simulink model "PID_Insuline_and_Glucogen"  (R2017b)
settings: Solver=ode45  StartTime=0.0  StopTime=18000  RelTol=1e-3
libraries: simulink x5
settings Model: Creator=Nandhini . S  LastModifiedBy=Sunil

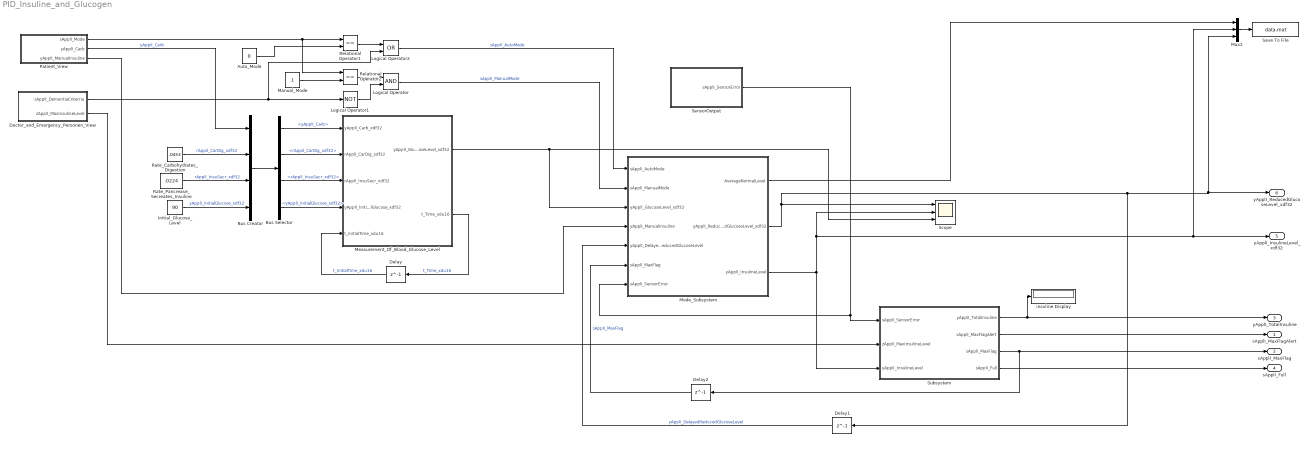
== system PID_Insuline_and_Glucogen ==
  Auto_Mode : Constant  Value=0
  Bus Creator : BusCreator  Inputs=4
  Bus Selector : BusSelector  OutputSignals=yApplI_Carb,rApplI_CarDig_xdf32,rApplI_InsuSecr_xdf32,yApplI_InitialGlucose_xdf32
  Delay : Delay  DelayLength=1  InitialCondition=0  SampleTime=60
  Delay1 : Delay  DelayLength=1  InitialCondition=0  SampleTime=1
  Delay2 : Delay  DelayLength=1  InitialCondition=0  SampleTime=1
  Doctor_and_Emergency_Personen_View : Subsystem
  Initial_Glucose_Level : Constant  Value=90
  Logical Operator : Logic  AllPortsSameDT=off  OutDataTypeStr=boolean
  Logical Operator1 : Logic  Operator=NOT  AllPortsSameDT=off  OutDataTypeStr=boolean
  Logical Operator2 : Logic  Operator=OR  AllPortsSameDT=off  OutDataTypeStr=boolean
  Manual_Mode : Constant
  Measurement_Of_Blood_Glucose_Level : Subsystem
  Mode_Subsystem : Subsystem
  Mux2 : Mux  Inputs=3
  Patient_View : Subsystem
  Rate_Carbohydrates_Digestion : Constant  Value=.0453
  Rate_Pancrease_Secreates_Insuline : Constant  Value=.0224
  Relational Operator1 : RelationalOperator  Operator===  OutDataTypeStr=boolean  RndMeth=Simplest
  Relational Operator2 : RelationalOperator  Operator===  OutDataTypeStr=boolean  RndMeth=Simplest
  Save To File : ToFile  Filename=data.mat  MatrixName=diabetic
  Scope : Scope  NumInputPorts=3
  SensorOutput : Subsystem
  Subsystem : Subsystem
  insuline Display : Display
  sApplI_MaxFlagAlert : Outport
  sApplI_MaxFlag : Outport  Port=2
  yApplI_TotalInsuline : Outport  Port=3
  sApplI_Full : Outport  Port=4
  yApplI_InsulineLevel_xdf32 : Outport  Port=5
  yApplI_ReducedGlucoseLevel_xdf32 : Outport  Port=6  InitialOutput=[0]
  wires:
  Bus Selector/4 -> Measurement_Of_Blood_Glucose_Level/4(yApplI_InitialGlucose_xdf32)  "<yApplI_InitialGlucose_xdf32>"
  Bus Selector/1 -> Measurement_Of_Blood_Glucose_Level/1(yApplI_Carb_xdf32)  "<yApplI_Carb>"
  Bus Creator/1 -> Bus Selector/1
  Bus Selector/2 -> Measurement_Of_Blood_Glucose_Level/2(rApplI_CarDig_xdf32)  "<rApplI_CarDig_xdf32>"
  Initial_Glucose_Level/1 -> Bus Creator/4  "yApplI_InitialGlucose_xdf32"
  Bus Selector/3 -> Measurement_Of_Blood_Glucose_Level/3(rApplI_InsuSecr_xdf32)  "<rApplI_InsuSecr_xdf32>"
  Rate_Pancrease_Secreates_Insuline/1 -> Bus Creator/3  "rApplI_InsuSecr_xdf32"
  Rate_Carbohydrates_Digestion/1 -> Bus Creator/2  "rApplI_CarDig_xdf32"
  Patient_View/2(yApplI_Carb) -> Bus Creator/1  "yApplI_Carb"
  Measurement_Of_Blood_Glucose_Level/1(yApplI_GlucoseLevel_xdf32) -> Mode_Subsystem/3(yApplI_GlucoseLevel_xdf32), Scope/3
  Relational Operator2/1 -> Logical Operator/1
  Auto_Mode/1 -> Relational Operator1/2
  Logical Operator1/1 -> Logical Operator/2
  Manual_Mode/1 -> Relational Operator2/2
  Relational Operator1/1 -> Logical Operator2/1
  Patient_View/1(sApplI_Mode) -> Relational Operator2/1, Relational Operator1/1
  Doctor_and_Emergency_Personen_View/1(sApplI_DementiaCriterria) -> Logical Operator2/2, Logical Operator1/1
  Doctor_and_Emergency_Personen_View/2(zApplI_MaxInsulineLevel) -> Subsystem/2(zApplI_MaxInsulineLevel)
  Subsystem/2(sApplI_MaxFlagAlert) -> sApplI_MaxFlagAlert/1
  Subsystem/3(sApplI_MaxFlag) -> Delay2/1, sApplI_MaxFlag/1
  Logical Operator2/1 -> Mode_Subsystem/1(sApplI_AutoMode)  "sApplI_AutoMode"
  Logical Operator/1 -> Mode_Subsystem/2(sApplI_ManualMode)  "sApplI_ManualMode"
  Patient_View/3(yApplI_ManualInsuline) -> Mode_Subsystem/4(yApplI_ManualInsuline)
  Mode_Subsystem/3(yApplI_InsulineLevel) -> Subsystem/3(yApplI_InsulineLevel), Mux2/2, yApplI_InsulineLevel_xdf32/1, Scope/2
  Mode_Subsystem/2(yApplI_ReducedGlucoseLevel_xdf32) -> Mux2/3, yApplI_ReducedGlucoseLevel_xdf32/1, Delay1/1, Scope/1
  Subsystem/1(yApplI_TotalInsuline) -> insuline Display/1, yApplI_TotalInsuline/1
  Subsystem/4(sApplI_Full) -> sApplI_Full/1
  SensorOutput/1(sApplI_SensorError) -> Mode_Subsystem/7(sApplI_SensorError), Subsystem/1(sApplI_SensorError)
  Mux2/1 -> Save To File/1
  Mode_Subsystem/1(AverageNormalLevel) -> Mux2/1
  Delay1/1 -> Mode_Subsystem/5(yApplI_DelayedReducedGlucoseLevel)  "yApplI_DelayedReducedGlucoseLevel"
  Measurement_Of_Blood_Glucose_Level/2(t_Time_xdu16) -> Delay/1  "t_Time_xdu16"
  Delay/1 -> Measurement_Of_Blood_Glucose_Level/5(t_InitialTime_xdu16)  "t_InitialTime_xdu16"
  Delay2/1 -> Mode_Subsystem/6(sApplI_MaxFlag)  "sApplI_MaxFlag"

== system PID_Insuline_and_Glucogen/Doctor_and_Emergency_Personen_View ==
  Dementia_Criteria : Constant  Value=0
  Man_Insuline_Level : Constant  Value=30000
  sApplI_DementiaCriterria : Outport
  zApplI_MaxInsulineLevel : Outport  Port=2
  wires:
  Dementia_Criteria/1 -> sApplI_DementiaCriterria/1  "sApplI_DementiaCriterria"
  Man_Insuline_Level/1 -> zApplI_MaxInsulineLevel/1  "zApplI_MaxInsulineLevel"

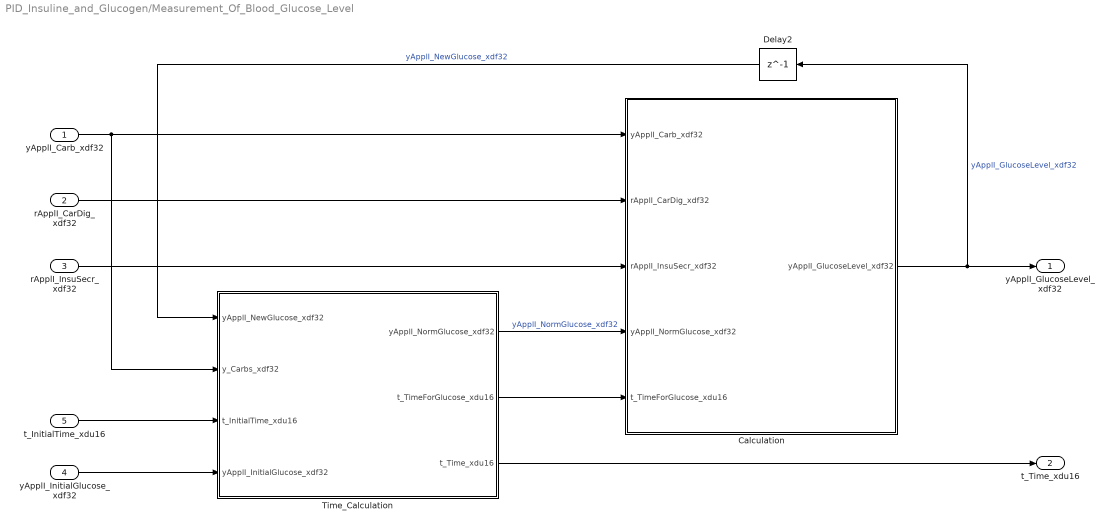
== system PID_Insuline_and_Glucogen/Measurement_Of_Blood_Glucose_Level ==
  yApplI_Carb_xdf32 : Inport
  rApplI_CarDig_xdf32 : Inport  Port=2
  rApplI_InsuSecr_xdf32 : Inport  Port=3
  yApplI_InitialGlucose_xdf32 : Inport  Port=4
  t_InitialTime_xdu16 : Inport  Port=5
  Calculation : Subsystem
  Delay2 : Delay  DelayLength=1  InitialCondition=0  SampleTime=60
  Time_Calculation : Subsystem
  yApplI_GlucoseLevel_xdf32 : Outport
  t_Time_xdu16 : Outport  Port=2
  wires:
  yApplI_Carb_xdf32/1 -> Calculation/1(yApplI_Carb_xdf32), Time_Calculation/2(y_Carbs_xdf32)
  rApplI_CarDig_xdf32/1 -> Calculation/2(rApplI_CarDig_xdf32)
  rApplI_InsuSecr_xdf32/1 -> Calculation/3(rApplI_InsuSecr_xdf32)
  t_InitialTime_xdu16/1 -> Time_Calculation/3(t_InitialTime_xdu16)
  Time_Calculation/3(t_Time_xdu16) -> t_Time_xdu16/1
  Calculation/1(yApplI_GlucoseLevel_xdf32) -> Delay2/1, yApplI_GlucoseLevel_xdf32/1  "yApplI_GlucoseLevel_xdf32"
  Delay2/1 -> Time_Calculation/1(yApplI_NewGlucose_xdf32)  "yApplI_NewGlucose_xdf32"
  Time_Calculation/2(t_TimeForGlucose_xdu16) -> Calculation/5(t_TimeForGlucose_xdu16)
  yApplI_InitialGlucose_xdf32/1 -> Time_Calculation/4(yApplI_InitialGlucose_xdf32)
  Time_Calculation/1(yApplI_NormGlucose_xdf32) -> Calculation/4(yApplI_NormGlucose_xdf32)  "yApplI_NormGlucose_xdf32"

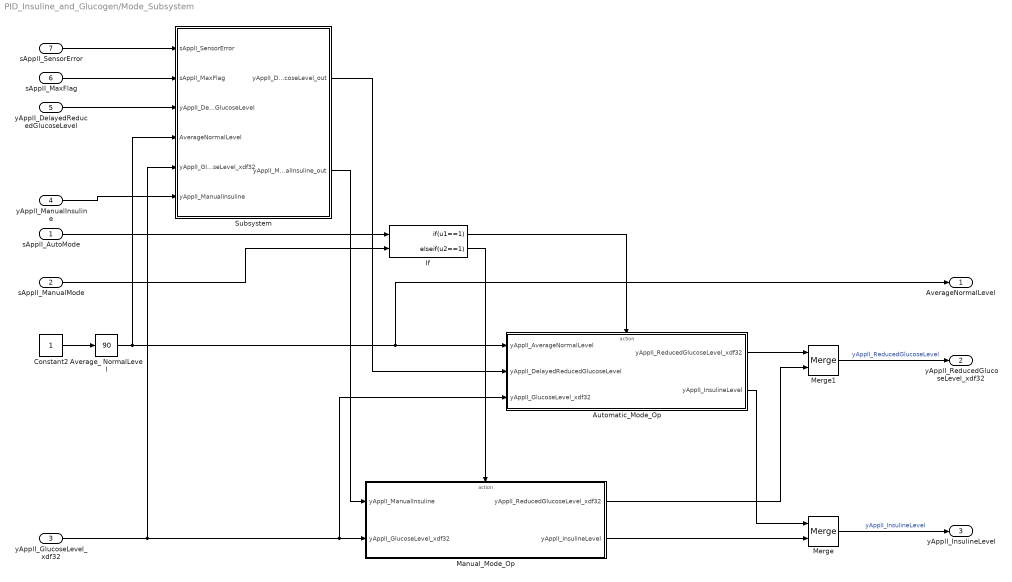
== system PID_Insuline_and_Glucogen/Mode_Subsystem ==
  sApplI_AutoMode : Inport
  sApplI_ManualMode : Inport  Port=2
  yApplI_GlucoseLevel_xdf32 : Inport  Port=3
  yApplI_ManualInsuline : Inport  Port=4
  yApplI_DelayedReducedGlucoseLevel : Inport  Port=5
  sApplI_MaxFlag : Inport  Port=6
  sApplI_SensorError : Inport  Port=7
  Automatic_Mode_Op : Subsystem
  Average_ NormalLevel : simulink/Math Operations/Slider Gain  gain=90  low=50  high=120
  Constant2 : Constant
  If : If  NumInputs=2  IfExpression=u1==1  ElseIfExpressions=u2==1  ShowElse=off  ZeroCross=off
  Manual_Mode_Op : Subsystem
  Merge : Merge
  Merge1 : Merge
  Subsystem : Subsystem
  AverageNormalLevel : Outport
  yApplI_ReducedGlucoseLevel_xdf32 : Outport  Port=2
  yApplI_InsulineLevel : Outport  Port=3
  wires:
  yApplI_GlucoseLevel_xdf32/1 -> Subsystem/5(yApplI_GlucoseLevel_xdf32), Automatic_Mode_Op/3(yApplI_GlucoseLevel_xdf32), Manual_Mode_Op/2(yApplI_GlucoseLevel_xdf32)
  Average_ NormalLevel/1 -> Subsystem/4(AverageNormalLevel), AverageNormalLevel/1, Automatic_Mode_Op/1(yApplI_AverageNormalLevel)
  sApplI_ManualMode/1 -> If/2
  Merge1/1 -> yApplI_ReducedGlucoseLevel_xdf32/1  "yApplI_ReducedGlucoseLevel"
  Automatic_Mode_Op/1(yApplI_ReducedGlucoseLevel_xdf32) -> Merge1/1
  Manual_Mode_Op/1(yApplI_ReducedGlucoseLevel_xdf32) -> Merge1/2
  If/2 -> Manual_Mode_Op/Action
  Manual_Mode_Op/2(yApplI_InsulineLevel) -> Merge/2
  If/1 -> Automatic_Mode_Op/Action
  Automatic_Mode_Op/2(yApplI_InsulineLevel) -> Merge/1
  Merge/1 -> yApplI_InsulineLevel/1  "yApplI_InsulineLevel"
  yApplI_ManualInsuline/1 -> Subsystem/6(yApplI_ManualInsuline)
  Constant2/1 -> Average_ NormalLevel/1
  yApplI_DelayedReducedGlucoseLevel/1 -> Subsystem/3(yApplI_DelayedReducedGlucoseLevel)
  sApplI_AutoMode/1 -> If/1
  sApplI_SensorError/1 -> Subsystem/1(sApplI_SensorError)
  sApplI_MaxFlag/1 -> Subsystem/2(sApplI_MaxFlag)
  Subsystem/1(yApplI_DelayedReducedGlucoseLevel_out) -> Automatic_Mode_Op/2(yApplI_DelayedReducedGlucoseLevel)
  Subsystem/2(yApplI_ManualInsuline_out) -> Manual_Mode_Op/1(yApplI_ManualInsuline)

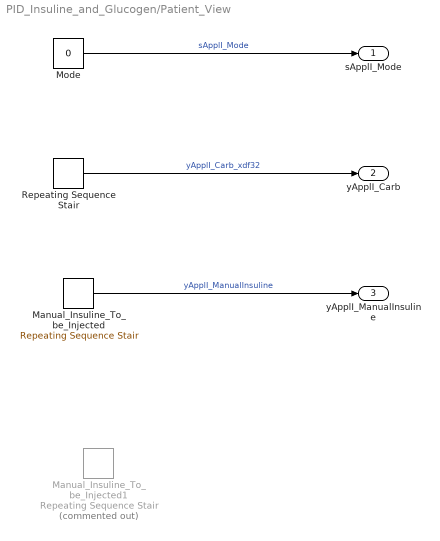
== system PID_Insuline_and_Glucogen/Patient_View ==
  Manual_Insuline_To_be_Injected : simulink/Sources/Repeating Sequence Stair  OutValues="[10 0 0 0  10 0 0 0 0 0 0 0 0 0 10 0 0 ].'"  tsamp=1000  OutMin=[]  OutMax=[]  OutDataTypeStr=double  OutputDataTypeScalingMode=double  OutDataType=fixdt(0,8)  ConRadixGroup=Best Precision: Vector-wise  OutScaling=2^-12
  Manual_Insuline_To_be_Injected1 : simulink/Sources/Repeating Sequence Stair  Commented=on  OutValues=[1 0 0 0 1 1 0 0 0 0 1 1 0 0 0 1 0 0 ].'  tsamp=1000  OutMin=[]  OutMax=[]  OutDataTypeStr=double  OutputDataTypeScalingMode=double  OutDataType=fixdt(0,8)  ConRadixGroup=Best Precision: Vector-wise  OutScaling=2^-12
  Mode : Constant  Value=0
  Repeating Sequence Stair : simulink/Sources/Repeating Sequence Stair  OutValues=[500 40 200 210 300 160].'  tsamp=3000  OutMin=[]  OutMax=[]  OutDataTypeStr=double  OutputDataTypeScalingMode=double  OutDataType=fixdt(0,8)  ConRadixGroup=Best Precision: Vector-wise  OutScaling=2^-12
  sApplI_Mode : Outport
  yApplI_Carb : Outport  Port=2
  yApplI_ManualInsuline : Outport  Port=3
  wires:
  Mode/1 -> sApplI_Mode/1  "sApplI_Mode"
  Repeating Sequence Stair/1 -> yApplI_Carb/1  "yApplI_Carb_xdf32"
  Manual_Insuline_To_be_Injected/1 -> yApplI_ManualInsuline/1  "yApplI_ManualInsuline"

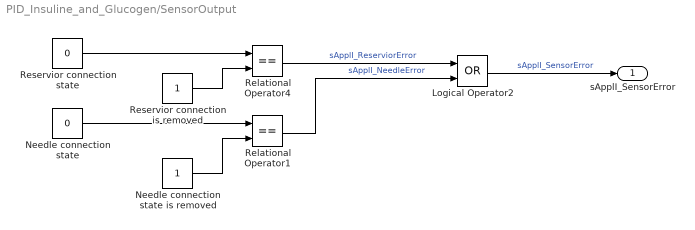
== system PID_Insuline_and_Glucogen/SensorOutput ==
  Logical Operator2 : Logic  Operator=OR  AllPortsSameDT=off  OutDataTypeStr=boolean
  Needle connection state : Constant  Value=0
  Needle connection state is removed : Constant
  Relational Operator1 : RelationalOperator  Operator===  OutDataTypeStr=boolean  RndMeth=Simplest
  Relational Operator4 : RelationalOperator  Operator===  OutDataTypeStr=boolean  RndMeth=Simplest
  Reservior connection is removed : Constant
  Reservior connection state : Constant  Value=0
  sApplI_SensorError : Outport
  wires:
  Reservior connection state/1 -> Relational Operator4/1
  Reservior connection is removed/1 -> Relational Operator4/2
  Needle connection state/1 -> Relational Operator1/1
  Needle connection state is removed/1 -> Relational Operator1/2
  Relational Operator4/1 -> Logical Operator2/1  "sApplI_ReserviorError"
  Relational Operator1/1 -> Logical Operator2/2  "sApplI_NeedleError"
  Logical Operator2/1 -> sApplI_SensorError/1  "sApplI_SensorError"

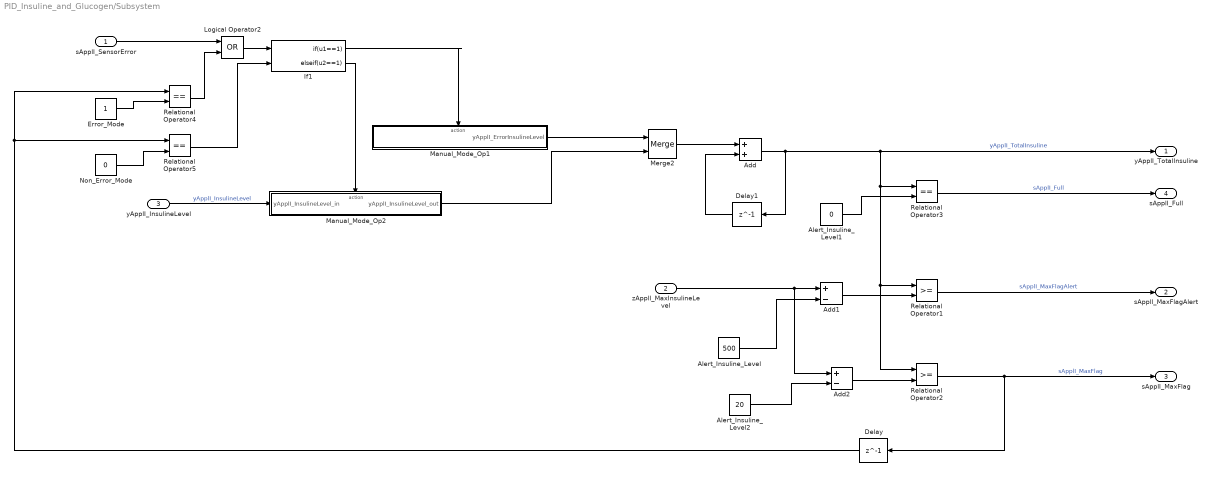
== system PID_Insuline_and_Glucogen/Subsystem ==
  sApplI_SensorError : Inport
  zApplI_MaxInsulineLevel : Inport  Port=2
  yApplI_InsulineLevel : Inport  Port=3
  Add : Sum
  Add1 : Sum  Inputs=+-
  Add2 : Sum  Inputs=+-
  Alert_Insuline_Level : Constant  Value=500
  Alert_Insuline_Level1 : Constant  Value=0
  Alert_Insuline_Level2 : Constant  Value=20
  Delay : Delay  DelayLength=1  InitialCondition=0
  Delay1 : Delay  DelayLength=1  InitialCondition=0  SampleTime=1
  Error_Mode : Constant
  If1 : If  NumInputs=2  IfExpression=u1==1  ElseIfExpressions=u2==1  ShowElse=off
  Logical Operator2 : Logic  Operator=OR  AllPortsSameDT=off  OutDataTypeStr=boolean
  Manual_Mode_Op1 : Subsystem
  Manual_Mode_Op2 : Subsystem
  Merge2 : Merge
  Non_Error_Mode : Constant  Value=0
  Relational Operator1 : RelationalOperator  OutDataTypeStr=boolean  RndMeth=Simplest
  Relational Operator2 : RelationalOperator  OutDataTypeStr=boolean  RndMeth=Simplest
  Relational Operator3 : RelationalOperator  Operator===  OutDataTypeStr=boolean  RndMeth=Simplest
  Relational Operator4 : RelationalOperator  Operator===  OutDataTypeStr=boolean  RndMeth=Simplest
  Relational Operator5 : RelationalOperator  Operator===  OutDataTypeStr=boolean  RndMeth=Simplest
  yApplI_TotalInsuline : Outport
  sApplI_MaxFlagAlert : Outport  Port=2
  sApplI_MaxFlag : Outport  Port=3
  sApplI_Full : Outport  Port=4
  wires:
  Delay1/1 -> Add/2
  Add/1 -> Delay1/1, Relational Operator3/1, Relational Operator2/1, Relational Operator1/1, yApplI_TotalInsuline/1  "yApplI_TotalInsuline"
  Merge2/1 -> Add/1
  zApplI_MaxInsulineLevel/1 -> Add2/1, Add1/1
  Alert_Insuline_Level/1 -> Add1/2
  Add1/1 -> Relational Operator1/2
  Relational Operator1/1 -> sApplI_MaxFlagAlert/1  "sApplI_MaxFlagAlert"
  Relational Operator2/1 -> Delay/1, sApplI_MaxFlag/1  "sApplI_MaxFlag"
  Alert_Insuline_Level1/1 -> Relational Operator3/2
  Relational Operator3/1 -> sApplI_Full/1  "sApplI_Full"
  Relational Operator5/1 -> If1/2
  Error_Mode/1 -> Relational Operator4/2
  Relational Operator4/1 -> Logical Operator2/2
  Delay/1 -> Relational Operator5/1, Relational Operator4/1
  Non_Error_Mode/1 -> Relational Operator5/2
  If1/1 -> Manual_Mode_Op1/Action
  If1/2 -> Manual_Mode_Op2/Action
  Manual_Mode_Op1/1(yApplI_ErrorInsulineLevel) -> Merge2/1
  yApplI_InsulineLevel/1 -> Manual_Mode_Op2/1(yApplI_InsulineLevel_in)  "yApplI_InsulineLevel"
  Manual_Mode_Op2/1(yApplI_InsulineLevel_out) -> Merge2/2
  Logical Operator2/1 -> If1/1
  sApplI_SensorError/1 -> Logical Operator2/1
  Alert_Insuline_Level2/1 -> Add2/2
  Add2/1 -> Relational Operator2/2

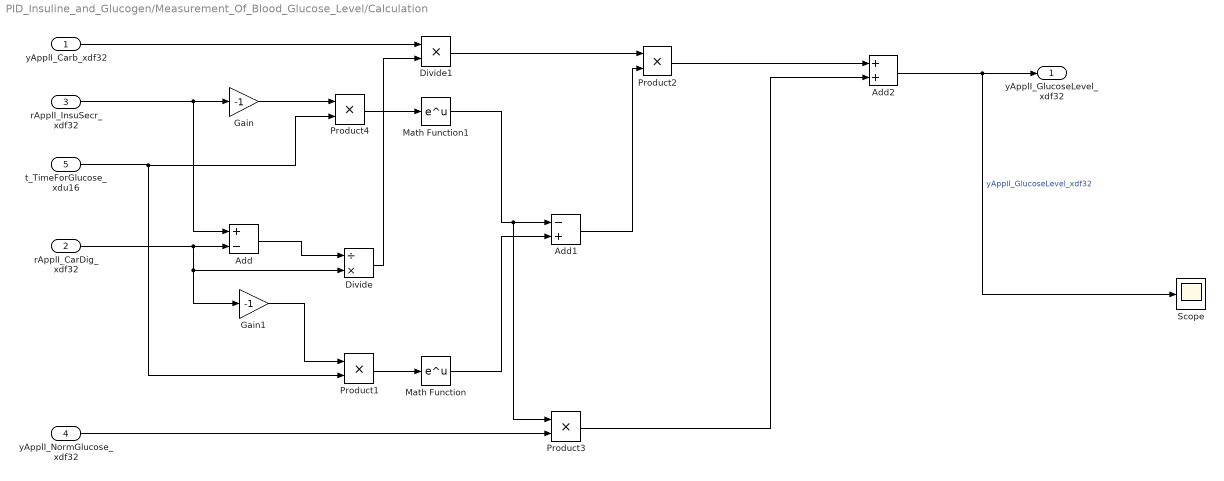
== system PID_Insuline_and_Glucogen/Measurement_Of_Blood_Glucose_Level/Calculation ==
  yApplI_Carb_xdf32 : Inport
  rApplI_CarDig_xdf32 : Inport  Port=2
  rApplI_InsuSecr_xdf32 : Inport  Port=3
  yApplI_NormGlucose_xdf32 : Inport  Port=4
  t_TimeForGlucose_xdu16 : Inport  Port=5
  Add : Sum  Inputs=+-
  Add1 : Sum  Inputs=-+  OutDataTypeStr=double
  Add2 : Sum
  Divide : Product  Inputs=/*
  Divide1 : Product  Inputs=**
  Gain : Gain  Gain=-1
  Gain1 : Gain  Gain=-1
  Math Function : Math  SaturateOnIntegerOverflow=on
  Math Function1 : Math  SaturateOnIntegerOverflow=on
  Product{1..4} (4 alike) : Product
  Scope : Scope
  yApplI_GlucoseLevel_xdf32 : Outport
  wires:
  rApplI_CarDig_xdf32/1 -> Add/2, Gain1/1, Divide/2
  rApplI_InsuSecr_xdf32/1 -> Add/1, Gain/1
  yApplI_NormGlucose_xdf32/1 -> Product3/2
  yApplI_Carb_xdf32/1 -> Divide1/1
  Add/1 -> Divide/1
  Divide/1 -> Divide1/2
  Gain1/1 -> Product1/1
  t_TimeForGlucose_xdu16/1 -> Product4/2, Product1/2
  Gain/1 -> Product4/1
  Product1/1 -> Math Function/1
  Math Function1/1 -> Product3/1, Add1/1
  Math Function/1 -> Add1/2
  Add1/1 -> Product2/2
  Divide1/1 -> Product2/1
  Product2/1 -> Add2/1
  Add2/1 -> Scope/1, yApplI_GlucoseLevel_xdf32/1  "yApplI_GlucoseLevel_xdf32"
  Product4/1 -> Math Function1/1
  Product3/1 -> Add2/2

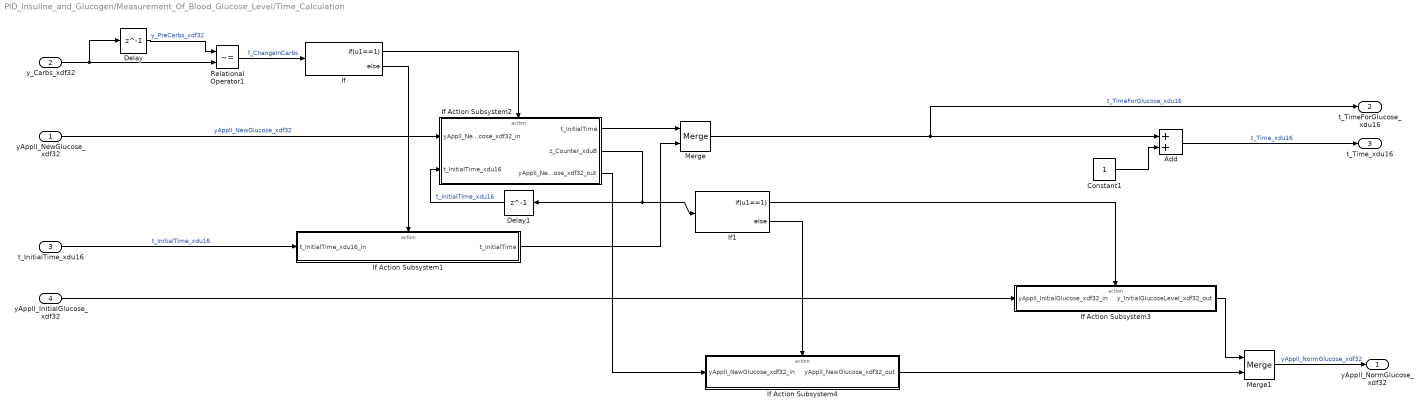
== system PID_Insuline_and_Glucogen/Measurement_Of_Blood_Glucose_Level/Time_Calculation ==
  yApplI_NewGlucose_xdf32 : Inport
  y_Carbs_xdf32 : Inport  Port=2
  t_InitialTime_xdu16 : Inport  Port=3
  yApplI_InitialGlucose_xdf32 : Inport  Port=4
  Add : Sum
  Constant1 : Constant
  Delay : Delay  DelayLength=1  InitialCondition=0  SampleTime=60
  Delay1 : Delay  DelayLength=1  InitialCondition=0  SampleTime=60
  If : If  IfExpression=u1==1
  If Action Subsystem1 : Subsystem  TreatAsAtomicUnit=on
  If Action Subsystem2 : Subsystem  TreatAsAtomicUnit=on
  If Action Subsystem3 : Subsystem  TreatAsAtomicUnit=on
  If Action Subsystem4 : Subsystem  TreatAsAtomicUnit=on
  If1 : If  IfExpression=u1==1
  Merge : Merge
  Merge1 : Merge
  Relational Operator1 : RelationalOperator  Operator=~=  OutDataTypeStr=boolean  RndMeth=Simplest
  yApplI_NormGlucose_xdf32 : Outport
  t_TimeForGlucose_xdu16 : Outport  Port=2
  t_Time_xdu16 : Outport  Port=3
  wires:
  If/2 -> If Action Subsystem1/Action
  Merge/1 -> Add/1, t_TimeForGlucose_xdu16/1  "t_TimeForGlucose_xdu16"
  t_InitialTime_xdu16/1 -> If Action Subsystem1/1(t_InitialTime_xdu16_in)  "t_InitialTime_xdu16"
  y_Carbs_xdf32/1 -> Delay/1, Relational Operator1/2
  Delay/1 -> Relational Operator1/1  "y_PreCarbs_xdf32"
  If/1 -> If Action Subsystem2/Action
  If Action Subsystem2/1(t_InitialTime) -> Merge/1
  Constant1/1 -> Add/2
  Add/1 -> t_Time_xdu16/1  "t_Time_xdu16"
  If Action Subsystem1/1(t_InitialTime) -> Merge/2
  Relational Operator1/1 -> If/1  "f_ChangeInCarbs"
  If Action Subsystem2/2(z_Counter_xdu8) -> Delay1/1, If1/1
  Delay1/1 -> If Action Subsystem2/2(t_InitialTime_xdu16)  "t_InitialTime_xdu16"
  If1/1 -> If Action Subsystem3/Action
  If1/2 -> If Action Subsystem4/Action
  yApplI_InitialGlucose_xdf32/1 -> If Action Subsystem3/1(yApplI_InitialGlucose_xdf32_in)
  If Action Subsystem3/1(y_InitialGlucoseLevel_xdf32_out) -> Merge1/1
  Merge1/1 -> yApplI_NormGlucose_xdf32/1  "yApplI_NormGlucose_xdf32"
  If Action Subsystem2/3(yApplI_NewGlucose_xdf32_out) -> If Action Subsystem4/1(yApplI_NewGlucose_xdf32_in)
  yApplI_NewGlucose_xdf32/1 -> If Action Subsystem2/1(yApplI_NewGlucose_xdf32_in)  "yApplI_NewGlucose_xdf32"
  If Action Subsystem4/1(yApplI_NewGlucose_xdf32_out) -> Merge1/2

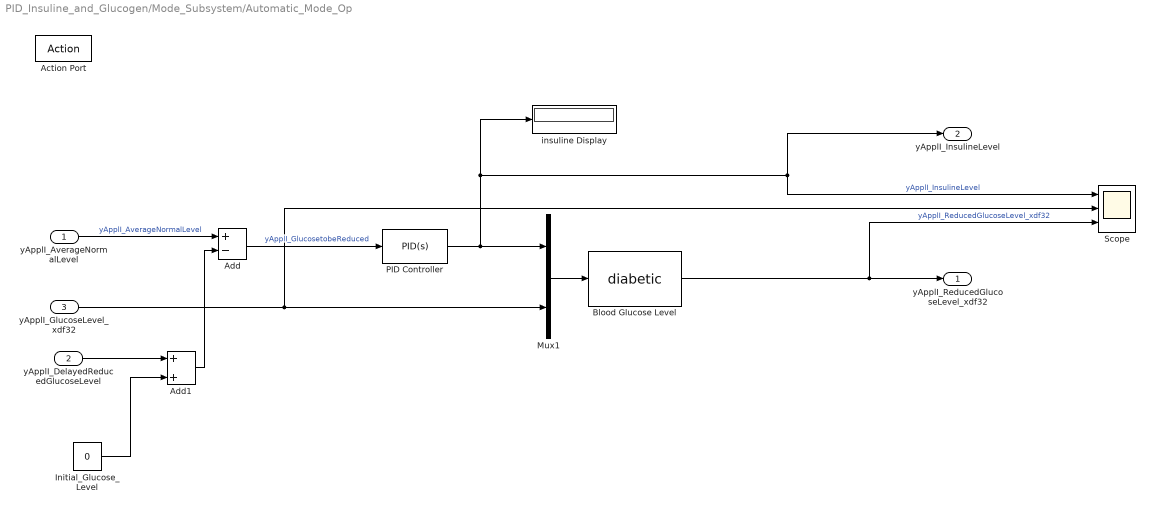
== system PID_Insuline_and_Glucogen/Mode_Subsystem/Automatic_Mode_Op ==
  yApplI_AverageNormalLevel : Inport
  yApplI_DelayedReducedGlucoseLevel : Inport  Port=2
  yApplI_GlucoseLevel_xdf32 : Inport  Port=3
  Action Port : ActionPort  ActionType=then
  Add : Sum  Inputs=+-
  Add1 : Sum
  Blood Glucose Level : S-Function  FunctionName=diabetic  SFunctionDeploymentMode=off  EnableBusSupport=off
  Initial_Glucose_Level : Constant  Value=0
  Mux1 : Mux  Inputs=2
  PID Controller : simulink/Continuous/PID Controller  Controller=PID  TimeDomain=Continuous-time  SampleTime=-1  IntegratorMethod=Forward Euler  FilterMethod=Forward Euler  Form=Parallel  UseFilter=on  ControllerParametersSource=internal  P=-0.05  I=-0.1  D=0  N=100  InitialConditionSource=internal  InitialConditionForIntegrator=3  InitialConditionForFilter=0  ExternalReset=none  LimitOutput=on  UpperSaturationLimit=10  LowerSaturationLimit=0  LinearizeAsGain=on  AntiWindupMode=back-calculation  Kb=1  TrackingMode=off  Kt=1  PParamMin=[]  PParamMax=[]  IParamMin=[]  IParamMax=[]  DParamMin=[]  DParamMax=[]  NParamMin=[]  NParamMax=[]  KbParamMin=[]  KbParamMax=[]  KtParamMin=[]  KtParamMax=[]  POutMin=[]  POutMax=[]  IOutMin=[]  IOutMax=[]  DOutMin=[]  DOutMax=[]  NOutMin=[]  NOutMax=[]  KbOutMin=[]  KbOutMax=[]  KtOutMin=[]  KtOutMax=[]  IntegratorOutMin=[]  IntegratorOutMax=[]  FilterOutMin=[]  FilterOutMax=[]  SumOutMin=[]  SumOutMax=[]  SumI1OutMin=[]  SumI1OutMax=[]  SumI2OutMin=[]  SumI2OutMax=[]  SumI3OutMin=[]  SumI3OutMax=[]  SumDOutMin=[]  SumDOutMax=[]  SaturationOutMin=[]  SaturationOutMax=[]  IntegratorContinuousStateAttributes=''  IntegratorStateMustResolveToSignalObject=off  IntegratorRTWStateStorageClass=Auto  FilterContinuousStateAttributes=''  FilterStateMustResolveToSignalObject=off  FilterRTWStateStorageClass=Auto  DifferentiatorICPrevScaledInput=0  DifferentiatorOutMin=[]  DifferentiatorOutMax=[]  InitialConditionSetting=State (most efficient)  FilterDiffOutCoefMin=[]  FilterDiffOutCoefMax=[]  SumDenOutMin=[]  SumDenOutMax=[]  SumNumOutMin=[]  SumNumOutMax=[]  ReciprocalOutMin=[]  ReciprocalOutMax=[]  DivideOutMin=[]  DivideOutMax=[]  TunerSelectOption=Transfer Function Based (PID Tuner App)
  Scope : Scope  NumInputPorts=3
  insuline Display : Display
  yApplI_ReducedGlucoseLevel_xdf32 : Outport  InitialOutput=[0]
  yApplI_InsulineLevel : Outport  Port=2
  wires:
  yApplI_GlucoseLevel_xdf32/1 -> Scope/2, Mux1/2
  yApplI_AverageNormalLevel/1 -> Add/1  "yApplI_AverageNormalLevel"
  Add/1 -> PID Controller/1  "yApplI_GlucosetobeReduced"
  Mux1/1 -> Blood Glucose Level/1
  PID Controller/1 -> yApplI_InsulineLevel/1, Scope/1, insuline Display/1, Mux1/1  "yApplI_InsulineLevel"
  Blood Glucose Level/1 -> yApplI_ReducedGlucoseLevel_xdf32/1, Scope/3  "yApplI_ReducedGlucoseLevel_xdf32"
  Initial_Glucose_Level/1 -> Add1/2
  Add1/1 -> Add/2
  yApplI_DelayedReducedGlucoseLevel/1 -> Add1/1

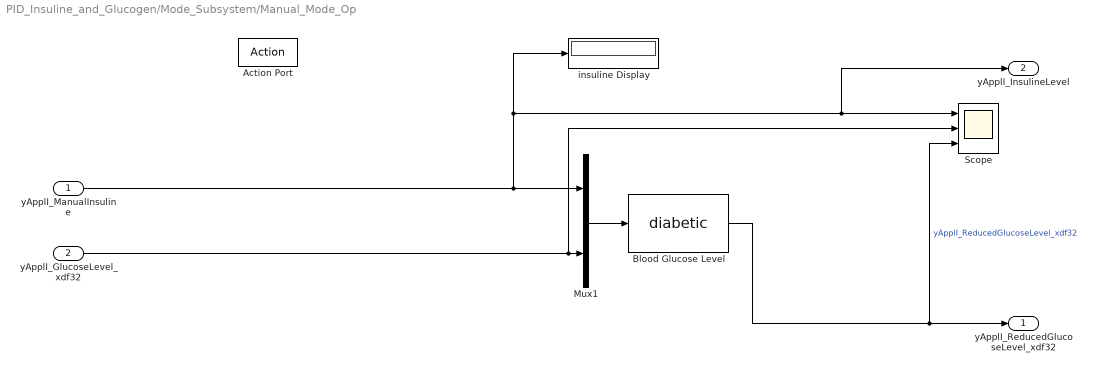
== system PID_Insuline_and_Glucogen/Mode_Subsystem/Manual_Mode_Op ==
  yApplI_ManualInsuline : Inport
  yApplI_GlucoseLevel_xdf32 : Inport  Port=2
  Action Port : ActionPort  ActionType=elseif
  Blood Glucose Level : S-Function  FunctionName=diabetic  SFunctionDeploymentMode=off  EnableBusSupport=off
  Mux1 : Mux  Inputs=2
  Scope : Scope  NumInputPorts=3
  insuline Display : Display
  yApplI_ReducedGlucoseLevel_xdf32 : Outport  InitialOutput=[0]
  yApplI_InsulineLevel : Outport  Port=2
  wires:
  yApplI_GlucoseLevel_xdf32/1 -> Mux1/2, Scope/2
  Mux1/1 -> Blood Glucose Level/1
  yApplI_ManualInsuline/1 -> yApplI_InsulineLevel/1, Scope/1, insuline Display/1, Mux1/1
  Blood Glucose Level/1 -> yApplI_ReducedGlucoseLevel_xdf32/1, Scope/3  "yApplI_ReducedGlucoseLevel_xdf32"

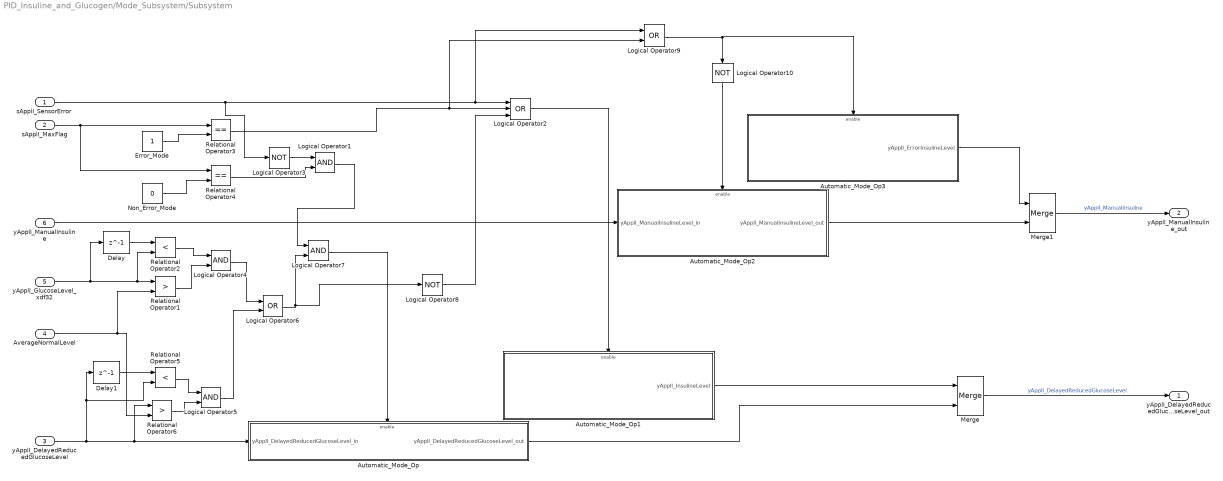
== system PID_Insuline_and_Glucogen/Mode_Subsystem/Subsystem ==
  sApplI_SensorError : Inport
  sApplI_MaxFlag : Inport  Port=2
  yApplI_DelayedReducedGlucoseLevel : Inport  Port=3
  AverageNormalLevel : Inport  Port=4
  yApplI_GlucoseLevel_xdf32 : Inport  Port=5
  yApplI_ManualInsuline : Inport  Port=6
  Automatic_Mode_Op : Subsystem
  Automatic_Mode_Op1 : Subsystem
  Automatic_Mode_Op2 : Subsystem
  Automatic_Mode_Op3 : Subsystem
  Delay : Delay  DelayLength=1  InitialCondition=0  SampleTime=60
  Delay1 : Delay  DelayLength=1  InitialCondition=0  SampleTime=60
  Error_Mode : Constant
  Logical Operator{1,4..5,7} (4 alike) : Logic  AllPortsSameDT=off  OutDataTypeStr=boolean
  Logical Operator10 : Logic  Operator=NOT  AllPortsSameDT=off  OutDataTypeStr=boolean
  Logical Operator2 : Logic  Operator=OR  Inputs=3  AllPortsSameDT=off  OutDataTypeStr=boolean
  Logical Operator3 : Logic  Operator=NOT  AllPortsSameDT=off  OutDataTypeStr=boolean
  Logical Operator6 : Logic  Operator=OR  AllPortsSameDT=off  OutDataTypeStr=boolean
  Logical Operator8 : Logic  Operator=NOT  AllPortsSameDT=off  OutDataTypeStr=boolean
  Logical Operator9 : Logic  Operator=OR  AllPortsSameDT=off  OutDataTypeStr=boolean
  Merge : Merge
  Merge1 : Merge
  Non_Error_Mode : Constant  Value=0
  Relational Operator1 : RelationalOperator  Operator=>  OutDataTypeStr=boolean  RndMeth=Simplest
  Relational Operator2 : RelationalOperator  Operator=<  OutDataTypeStr=boolean  RndMeth=Simplest
  Relational Operator3 : RelationalOperator  Operator===  OutDataTypeStr=boolean  RndMeth=Simplest
  Relational Operator4 : RelationalOperator  Operator===  OutDataTypeStr=boolean  RndMeth=Simplest
  Relational Operator5 : RelationalOperator  Operator=<  OutDataTypeStr=boolean  RndMeth=Simplest
  Relational Operator6 : RelationalOperator  Operator=>  OutDataTypeStr=boolean  RndMeth=Simplest
  yApplI_DelayedReducedGlucoseLevel_out : Outport
  yApplI_ManualInsuline_out : Outport  Port=2
  wires:
  Relational Operator3/1 -> Logical Operator9/2, Logical Operator2/2
  Non_Error_Mode/1 -> Relational Operator4/2
  sApplI_SensorError/1 -> Logical Operator3/1, Logical Operator9/1, Logical Operator2/1
  sApplI_MaxFlag/1 -> Relational Operator4/1, Relational Operator3/1
  Error_Mode/1 -> Relational Operator3/2
  yApplI_DelayedReducedGlucoseLevel/1 -> Relational Operator5/2, Delay1/1, Relational Operator6/1, Automatic_Mode_Op/1(yApplI_DelayedReducedGlucoseLevel_in)
  Relational Operator4/1 -> Logical Operator1/2
  Logical Operator2/1 -> Automatic_Mode_Op1/Enable
  Automatic_Mode_Op1/1(yApplI_InsulineLevel) -> Merge/1
  Automatic_Mode_Op/1(yApplI_DelayedReducedGlucoseLevel_out) -> Merge/2
  Merge/1 -> yApplI_DelayedReducedGlucoseLevel_out/1  "yApplI_DelayedReducedGlucoseLevel"
  Logical Operator3/1 -> Logical Operator1/1
  Logical Operator1/1 -> Logical Operator7/1
  yApplI_GlucoseLevel_xdf32/1 -> Delay/1, Relational Operator2/2, Relational Operator1/1
  AverageNormalLevel/1 -> Relational Operator6/2, Relational Operator1/2
  Delay/1 -> Relational Operator2/1
  Relational Operator2/1 -> Logical Operator4/1
  Relational Operator1/1 -> Logical Operator4/2
  Delay1/1 -> Relational Operator5/1
  Relational Operator5/1 -> Logical Operator5/1
  Relational Operator6/1 -> Logical Operator5/2
  Logical Operator4/1 -> Logical Operator6/1
  Logical Operator5/1 -> Logical Operator6/2
  Logical Operator6/1 -> Logical Operator8/1, Logical Operator7/2
  Logical Operator7/1 -> Automatic_Mode_Op/Enable
  Logical Operator8/1 -> Logical Operator2/3
  yApplI_ManualInsuline/1 -> Automatic_Mode_Op2/1(yApplI_ManualInsulineLevel_in)
  Automatic_Mode_Op3/1(yApplI_ErrorInsulineLevel) -> Merge1/1
  Automatic_Mode_Op2/1(yApplI_ManualInsulineLevel_out) -> Merge1/2
  Merge1/1 -> yApplI_ManualInsuline_out/1  "yApplI_ManualInsuline"
  Logical Operator9/1 -> Automatic_Mode_Op3/Enable, Logical Operator10/1
  Logical Operator10/1 -> Automatic_Mode_Op2/Enable

== system PID_Insuline_and_Glucogen/Subsystem/Manual_Mode_Op1 ==
  Action Port : ActionPort  ActionType=then
  Alert_Insuline_Level : Constant  Value=0
  yApplI_ErrorInsulineLevel : Outport
  wires:
  Alert_Insuline_Level/1 -> yApplI_ErrorInsulineLevel/1

== system PID_Insuline_and_Glucogen/Subsystem/Manual_Mode_Op2 ==
  yApplI_InsulineLevel_in : Inport
  Action Port : ActionPort  ActionType=elseif
  yApplI_InsulineLevel_out : Outport
  wires:
  yApplI_InsulineLevel_in/1 -> yApplI_InsulineLevel_out/1

== system PID_Insuline_and_Glucogen/Measurement_Of_Blood_Glucose_Level/Time_Calculation/If Action Subsystem1 ==
  t_InitialTime_xdu16_in : Inport
  Action Port : ActionPort  ActionType=else
  Add : Sum
  Constant : Constant
  t_InitialTime : Outport
  wires:
  t_InitialTime_xdu16_in/1 -> Add/1  "t_InitialTime_xdu16"
  Constant/1 -> Add/2
  Add/1 -> t_InitialTime/1  "t_InitialTime"

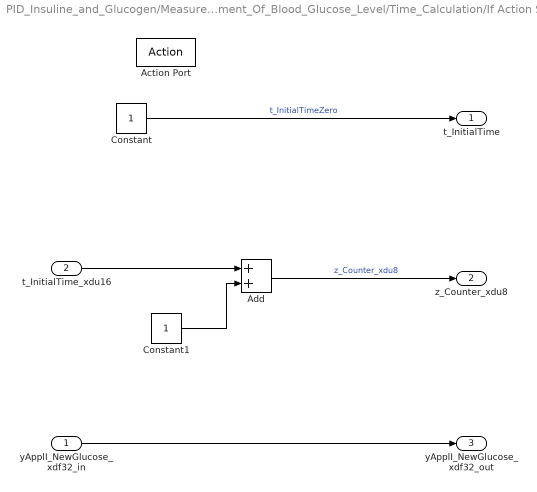
== system PID_Insuline_and_Glucogen/Measurement_Of_Blood_Glucose_Level/Time_Calculation/If Action Subsystem2 ==
  yApplI_NewGlucose_xdf32_in : Inport
  t_InitialTime_xdu16 : Inport  Port=2
  Action Port : ActionPort  ActionType=then
  Add : Sum
  Constant : Constant
  Constant1 : Constant
  t_InitialTime : Outport
  z_Counter_xdu8 : Outport  Port=2
  yApplI_NewGlucose_xdf32_out : Outport  Port=3
  wires:
  Constant/1 -> t_InitialTime/1  "t_InitialTimeZero"
  t_InitialTime_xdu16/1 -> Add/1
  Constant1/1 -> Add/2
  Add/1 -> z_Counter_xdu8/1  "z_Counter_xdu8"
  yApplI_NewGlucose_xdf32_in/1 -> yApplI_NewGlucose_xdf32_out/1

== system PID_Insuline_and_Glucogen/Measurement_Of_Blood_Glucose_Level/Time_Calculation/If Action Subsystem3 ==
  yApplI_InitialGlucose_xdf32_in : Inport
  Action Port : ActionPort  ActionType=then
  y_InitialGlucoseLevel_xdf32_out : Outport
  wires:
  yApplI_InitialGlucose_xdf32_in/1 -> y_InitialGlucoseLevel_xdf32_out/1

== system PID_Insuline_and_Glucogen/Measurement_Of_Blood_Glucose_Level/Time_Calculation/If Action Subsystem4 ==
  yApplI_NewGlucose_xdf32_in : Inport
  Action Port : ActionPort  ActionType=else
  yApplI_NewGlucose_xdf32_out : Outport
  wires:
  yApplI_NewGlucose_xdf32_in/1 -> yApplI_NewGlucose_xdf32_out/1

== system PID_Insuline_and_Glucogen/Mode_Subsystem/Subsystem/Automatic_Mode_Op ==
  yApplI_DelayedReducedGlucoseLevel_in : Inport
  Enable : EnablePort
  yApplI_DelayedReducedGlucoseLevel_out : Outport
  wires:
  yApplI_DelayedReducedGlucoseLevel_in/1 -> yApplI_DelayedReducedGlucoseLevel_out/1

== system PID_Insuline_and_Glucogen/Mode_Subsystem/Subsystem/Automatic_Mode_Op1 ==
  Enable : EnablePort
  Non_Error_Mode : Constant  Value=89
  yApplI_InsulineLevel : Outport
  wires:
  Non_Error_Mode/1 -> yApplI_InsulineLevel/1  "yApplI_AverageNormalLevel"

== system PID_Insuline_and_Glucogen/Mode_Subsystem/Subsystem/Automatic_Mode_Op2 ==
  yApplI_ManualInsulineLevel_in : Inport
  Enable : EnablePort
  yApplI_ManualInsulineLevel_out : Outport
  wires:
  yApplI_ManualInsulineLevel_in/1 -> yApplI_ManualInsulineLevel_out/1  "yApplI_ManualInsulineLevel"

== system PID_Insuline_and_Glucogen/Mode_Subsystem/Subsystem/Automatic_Mode_Op3 ==
  Enable : EnablePort
  Non_Error_Mode : Constant  Value=0
  yApplI_ErrorInsulineLevel : Outport  SampleTime=1000
  wires:
  Non_Error_Mode/1 -> yApplI_ErrorInsulineLevel/1  "yApplI_AverageNormalLevel"
